simulink model "dflipflop"  (R2020a)
settings: Solver=VariableStepAuto  StartTime=0.0  StopTime=10.0  RelTol=1e-3
libraries: simulink_extras x5
settings Model: Creator=F1  LastModifiedBy=F1

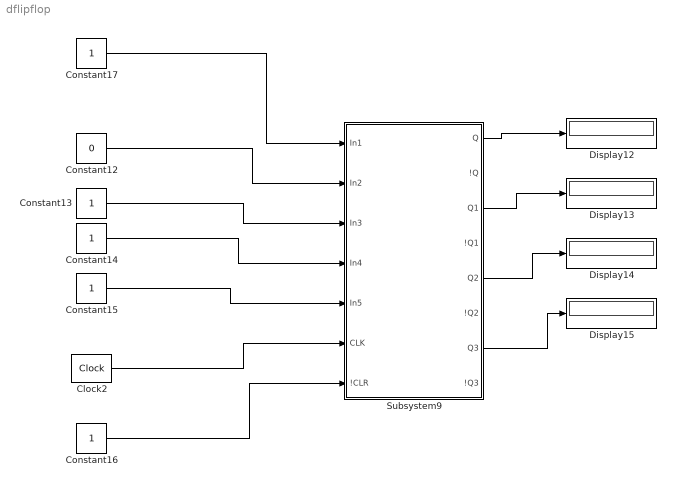
== system dflipflop ==
  Clock2 : simulink_extras/Flip Flops/Clock  period=2
  Constant12 : Constant  Value=0
  Constant{13..17} (5 alike) : Constant
  Display{12..15} (4 alike) : Display
  Subsystem9 : Subsystem
  wires:
  Subsystem9/5(Q2) -> Display14/1
  Subsystem9/7(Q3) -> Display15/1
  Subsystem9/3(Q1) -> Display13/1
  Constant14/1 -> Subsystem9/4(In4)
  Constant15/1 -> Subsystem9/5(In5)
  Constant13/1 -> Subsystem9/3(In3)
  Constant16/1 -> Subsystem9/7(!CLR)
  Constant12/1 -> Subsystem9/2(In2)
  Clock2/1 -> Subsystem9/6(CLK)
  Constant17/1 -> Subsystem9/1(In1)
  Subsystem9/1(Q) -> Display12/1

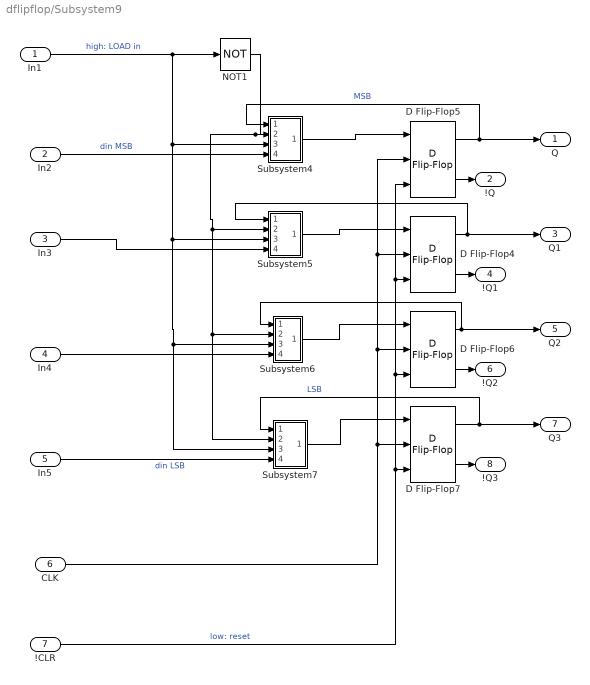
== system dflipflop/Subsystem9 ==
  In1 : Inport
  In2 : Inport  Port=2
  In3 : Inport  Port=3
  In4 : Inport  Port=4
  In5 : Inport  Port=5
  CLK : Inport  Port=6
  !CLR : Inport  Port=7
  D Flip-Flop{4..7} (4 alike) : simulink_extras/Flip Flops/D Flip-Flop
  NOT1 : Logic  Operator=NOT  IconShape=distinctive  AllPortsSameDT=off  OutDataTypeStr=boolean
  Subsystem4 : Subsystem
  Subsystem5 : Subsystem
  Subsystem6 : Subsystem
  Subsystem7 : Subsystem
  Q : Outport
  !Q : Outport  Port=2
  Q1 : Outport  Port=3
  !Q1 : Outport  Port=4
  Q2 : Outport  Port=5
  !Q2 : Outport  Port=6
  Q3 : Outport  Port=7
  !Q3 : Outport  Port=8
  wires:
  In5/1 -> Subsystem7/4(In4)  "din LSB"
  D Flip-Flop5/1 -> Q/1, Subsystem4/1(In1)  "MSB"
  NOT1/1 -> Subsystem7/2(In2), Subsystem6/2(In2), Subsystem5/2(In1), Subsystem4/2(In2)
  Subsystem4/1(Out1) -> D Flip-Flop5/1
  Subsystem7/1(Out1) -> D Flip-Flop7/1
  In3/1 -> Subsystem5/4(In4)
  D Flip-Flop4/2 -> !Q1/1
  D Flip-Flop4/1 -> Q1/1, Subsystem5/1(In2)
  D Flip-Flop7/2 -> !Q3/1
  D Flip-Flop7/1 -> Q3/1, Subsystem7/1(In1)  "LSB"
  D Flip-Flop5/2 -> !Q/1
  Subsystem5/1(Out1) -> D Flip-Flop4/1
  D Flip-Flop6/2 -> !Q2/1
  Subsystem6/1(Out1) -> D Flip-Flop6/1
  D Flip-Flop6/1 -> Q2/1, Subsystem6/1(In1)
  In1/1 -> Subsystem7/3(In3), Subsystem6/3(In3), Subsystem5/3(In3), Subsystem4/3(In3), NOT1/1  "high: LOAD in"
  !CLR/1 -> D Flip-Flop5/3, D Flip-Flop4/3, D Flip-Flop6/3, D Flip-Flop7/3  "low: reset"
  CLK/1 -> D Flip-Flop5/2, D Flip-Flop4/2, D Flip-Flop6/2, D Flip-Flop7/2
  In2/1 -> Subsystem4/4(In4)  "din MSB"
  In4/1 -> Subsystem6/4(In4)

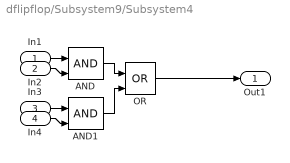
== system dflipflop/Subsystem9/Subsystem4 ==
  In1 : Inport
  In2 : Inport  Port=2
  In3 : Inport  Port=3
  In4 : Inport  Port=4
  AND : Logic  IconShape=distinctive  AllPortsSameDT=off  OutDataTypeStr=boolean
  AND1 : Logic  IconShape=distinctive  AllPortsSameDT=off  OutDataTypeStr=boolean
  OR : Logic  Operator=OR  IconShape=distinctive  AllPortsSameDT=off  OutDataTypeStr=boolean
  Out1 : Outport
  wires:
  AND/1 -> OR/1
  AND1/1 -> OR/2
  OR/1 -> Out1/1
  In3/1 -> AND1/1
  In4/1 -> AND1/2
  In2/1 -> AND/2
  In1/1 -> AND/1

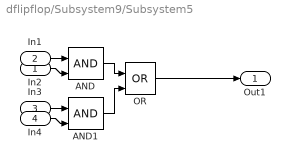
== system dflipflop/Subsystem9/Subsystem5 ==
  In2 : Inport
  In1 : Inport  Port=2
  In3 : Inport  Port=3
  In4 : Inport  Port=4
  AND : Logic  IconShape=distinctive  AllPortsSameDT=off  OutDataTypeStr=boolean
  AND1 : Logic  IconShape=distinctive  AllPortsSameDT=off  OutDataTypeStr=boolean
  OR : Logic  Operator=OR  IconShape=distinctive  AllPortsSameDT=off  OutDataTypeStr=boolean
  Out1 : Outport
  wires:
  AND/1 -> OR/1
  AND1/1 -> OR/2
  OR/1 -> Out1/1
  In3/1 -> AND1/1
  In4/1 -> AND1/2
  In2/1 -> AND/2
  In1/1 -> AND/1

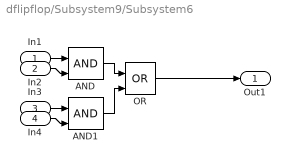
== system dflipflop/Subsystem9/Subsystem6 ==
  In1 : Inport
  In2 : Inport  Port=2
  In3 : Inport  Port=3
  In4 : Inport  Port=4
  AND : Logic  IconShape=distinctive  AllPortsSameDT=off  OutDataTypeStr=boolean
  AND1 : Logic  IconShape=distinctive  AllPortsSameDT=off  OutDataTypeStr=boolean
  OR : Logic  Operator=OR  IconShape=distinctive  AllPortsSameDT=off  OutDataTypeStr=boolean
  Out1 : Outport
  wires:
  AND/1 -> OR/1
  AND1/1 -> OR/2
  OR/1 -> Out1/1
  In3/1 -> AND1/1
  In4/1 -> AND1/2
  In2/1 -> AND/2
  In1/1 -> AND/1

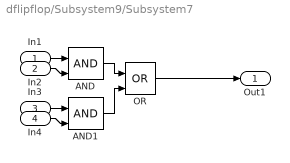
== system dflipflop/Subsystem9/Subsystem7 ==
  In1 : Inport
  In2 : Inport  Port=2
  In3 : Inport  Port=3
  In4 : Inport  Port=4
  AND : Logic  IconShape=distinctive  AllPortsSameDT=off  OutDataTypeStr=boolean
  AND1 : Logic  IconShape=distinctive  AllPortsSameDT=off  OutDataTypeStr=boolean
  OR : Logic  Operator=OR  IconShape=distinctive  AllPortsSameDT=off  OutDataTypeStr=boolean
  Out1 : Outport
  wires:
  AND/1 -> OR/1
  AND1/1 -> OR/2
  OR/1 -> Out1/1
  In3/1 -> AND1/1
  In4/1 -> AND1/2
  In2/1 -> AND/2
  In1/1 -> AND/1
